simulink model "bilant_masic"  (R2021a)
settings: Solver=VariableStepAuto  StartTime=0.0  StopTime=10.0  RelTol=1e-3
values from neighbouring files (symbols this model uses):
  c0 = 5.4698    [script.m]
  V = 10    [script.m]
settings Model: Creator=Automatica  LastModifiedBy=Automatica

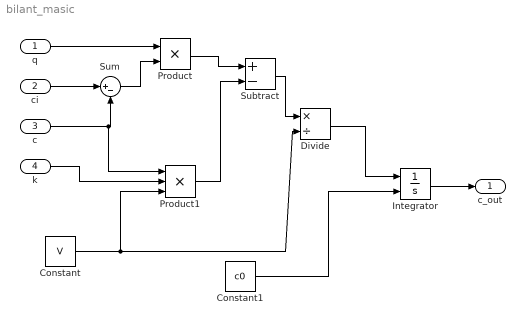
== system bilant_masic ==
  q : Inport
  ci : Inport  Port=2
  c : Inport  Port=3
  k : Inport  Port=4
  Constant : Constant  Value=V
  Constant1 : Constant  Value=c0
  Divide : Product  Inputs=*/
  Integrator : Integrator  InitialConditionSource=external
  Product : Product
  Product1 : Product  Inputs=3
  Subtract : Sum  Inputs=+-
  Sum : Sum  Inputs=|+-
  c_out : Outport
  wires:
  q/1 -> Product/1
  ci/1 -> Sum/1
  c/1 -> Sum/2, Product1/1
  k/1 -> Product1/2
  Constant/1 -> Divide/2, Product1/3
  Constant1/1 -> Integrator/2
  Sum/1 -> Product/2
  Product/1 -> Subtract/1
  Product1/1 -> Subtract/2
  Subtract/1 -> Divide/1
  Divide/1 -> Integrator/1
  Integrator/1 -> c_out/1
